simulink library "r2dbe_vdif_lib"  (R2012b)
settings: Solver=ode45  StartTime=0.0  StopTime=10.0  RelTol=1e-3
libraries: xbsIndex_r4 x360, casper_library_delays x11, casper_library_flow_control x3
(part 2 of 4)

== system r2dbe_vdif_lib/vdif/little_end ==
  sim_1 : Inport
  io_delay : xbsIndex_r4/Delay  rst=off  infoeditControl=Selection of Reset will increase slice count due to use of real FFs and instead of SRLs  en=off  latency=0  dbl_ovrd=off  reg_retiming=on  block_type=delay
  r2dbe_10gbe_f_vdif_little_end_user_data_out : xbsIndex_r4/Gateway In  gui_display_data_type=Fixed-point  arith_type=Unsigned  n_bits=32  bin_pt=0  preci_type=Single  exp_width=8  frac_width=24  quantization="Round  (unbiased: +/- Inf)"  overflow=Saturate  period=1  dbl_ovrd=off  timing_constraint=None  locs_specified=off  LOCs={}  UseAsADC=off  ADCChannel='1'  inherit_from_input=off  hdl_port=on  block_type=gatewayin
  reint1 : xbsIndex_r4/Reinterpret  force_arith_type=on  arith_type=Unsigned  force_bin_pt=on  bin_pt=0  block_type=reinterpret
  slice_reg : xbsIndex_r4/Slice  nbits=32  boolean_output=off  mode=Lower Bit Location + Width  bit1=0  base1=MSB of Input  bit0=0  base0=LSB of Input  dbl_ovrd=off  block_type=slice
  in_reg : Outport
  wires:
  reint1/1 -> in_reg/1
  slice_reg/1 -> reint1/1
  io_delay/1 -> slice_reg/1
  sim_1/1 -> r2dbe_10gbe_f_vdif_little_end_user_data_out/1
  r2dbe_10gbe_f_vdif_little_end_user_data_out/1 -> io_delay/1

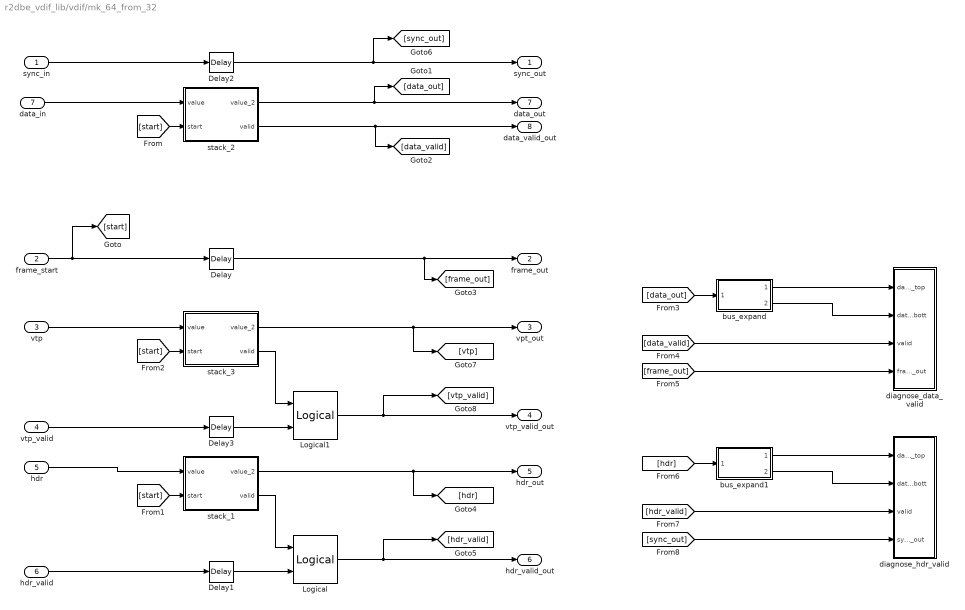
== system r2dbe_vdif_lib/vdif/mk_64_from_32 ==
  sync_in : Inport
  frame_start : Inport  Port=2
  vtp : Inport  Port=3
  vtp_valid : Inport  Port=4
  hdr : Inport  Port=5
  hdr_valid : Inport  Port=6
  data_in : Inport  Port=7
  Delay{,1..3} (4 alike) : xbsIndex_r4/Delay  rst=off  infoeditControl=Selection of Reset will increase slice count due to use of real FFs and instead of SRLs  en=off  latency=2  dbl_ovrd=off  reg_retiming=off  block_type=delay
  Logical : xbsIndex_r4/Logical  logical_function=AND  inputs=2  en=off  latency=0  precision=Full  arith_type=Unsigned  n_bits=16  bin_pt=0  align_bp=on  dbl_ovrd=off  block_type=logical
  Logical1 : xbsIndex_r4/Logical  logical_function=AND  inputs=2  en=off  latency=0  precision=Full  arith_type=Unsigned  n_bits=16  bin_pt=0  align_bp=on  dbl_ovrd=off  block_type=logical
  bus_expand : Subsystem  AncestorBlock=casper_library_flow_control/bus_expand  mask(bus_expand){mode=divisions of equal size, outputNum=2, outputWidth=32, outputBinaryPt=0, outputArithmeticType=0, show_format=off, outputToWorkspace=off, variablePrefix=out, outputToModelAsWell=on}
      mask prompts: outputNum "Number of outputs:"; outputWidth "Output width:"; outputBinaryPt "Output binary point position:"; outputArithmeticType "Output arithmetic type (ufix=0, fix=1, bool=2):"; show_format "Print format string?"; outputToWorkspace "Output to workspace?"; variablePrefix "Variable name prefix:"; outputToModelAsWell "Output to model as well?"
      mask help:
      | Expands a 'bus' made using a bus_create or Xilinx
      | concat block.
      | The input will be divided into the specified number
      | of outputs with the specified arithmetic types.
      | Divisions are made from most significant bit.
      mask init: same as r2dbe_vdif_lib/vdif/delay_data/bus_expand
      settings: AttributesFormatString=2 outputs
      mask TypeOptions mode: divisions of equal size | divisions of arbitrary size
      mask Callback mode: bus_expand_callback();
      mask Callback outputWidth: bus_expand_callback();
      mask Callback outputToWorkspace: bus_expand_callback();
  bus_expand1 : Subsystem  AncestorBlock=casper_library_flow_control/bus_expand  mask(bus_expand){mode=divisions of equal size, outputNum=2, outputWidth=32, outputBinaryPt=0, outputArithmeticType=0, show_format=off, outputToWorkspace=off, variablePrefix=out, outputToModelAsWell=on}
      mask prompts: outputNum "Number of outputs:"; outputWidth "Output width:"; outputBinaryPt "Output binary point position:"; outputArithmeticType "Output arithmetic type (ufix=0, fix=1, bool=2):"; show_format "Print format string?"; outputToWorkspace "Output to workspace?"; variablePrefix "Variable name prefix:"; outputToModelAsWell "Output to model as well?"
      mask help:
      | Expands a 'bus' made using a bus_create or Xilinx
      | concat block.
      | The input will be divided into the specified number
      | of outputs with the specified arithmetic types.
      | Divisions are made from most significant bit.
      mask init: same as r2dbe_vdif_lib/vdif/delay_data/bus_expand
      settings: AttributesFormatString=2 outputs
      mask TypeOptions mode: divisions of equal size | divisions of arbitrary size
      mask Callback mode: bus_expand_callback();
      mask Callback outputWidth: bus_expand_callback();
      mask Callback outputToWorkspace: bus_expand_callback();
  diagnose_data_valid : Subsystem
  diagnose_hdr_valid : Subsystem
  stack_1 : Subsystem
      mask help: stacks 2 samples together, based on a flag that indicates the start or the first sample of data to be stacked. outputs the stacked data and a valid signal, such that on any given valid signal the data represents the newest data in the top half and the oldest data in the lower half. Therefore given a data stream starting with 0, increasing by 1 every clock cycle I would expect the first data valid to indicate a piece of data with the value 0 in the low bits, 1 in the high, and the next sample having 2 in the low bits 3 in the high, etc.
  stack_2 : Subsystem
      mask help: stacks 2 samples together, based on a flag that indicates the start or the first sample of data to be stacked. outputs the stacked data and a valid signal, such that on any given valid signal the data represents the newest data in the top half and the oldest data in the lower half. Therefore given a data stream starting with 0, increasing by 1 every clock cycle I would expect the first data valid to indicate a piece of data with the value 0 in the low bits, 1 in the high, and the next sample having 2 in the low bits 3 in the high, etc.
  stack_3 : Subsystem
      mask help: stacks 2 samples together, based on a flag that indicates the start or the first sample of data to be stacked. outputs the stacked data and a valid signal, such that on any given valid signal the data represents the newest data in the top half and the oldest data in the lower half. Therefore given a data stream starting with 0, increasing by 1 every clock cycle I would expect the first data valid to indicate a piece of data with the value 0 in the low bits, 1 in the high, and the next sample having 2 in the low bits 3 in the high, etc.
  sync_out : Outport
  frame_out : Outport  Port=2
  vpt_out : Outport  Port=3
  vtp_valid_out : Outport  Port=4
  hdr_out : Outport  Port=5
  hdr_valid_out : Outport  Port=6
  data_out : Outport  Port=7
  data_valid_out : Outport  Port=8
  wires:
  hdr_valid/1 -> Delay1/1
  hdr/1 -> stack_1/1(value)
  vtp_valid/1 -> Delay3/1
  vtp/1 -> stack_3/1(value)
  Delay3/1 -> Logical1/2
  Logical1/1 -> [vtp_valid], vtp_valid_out/1
  stack_3/2(valid) -> Logical1/1
  stack_3/1(value_2) -> [vtp], vpt_out/1
  [start] -> stack_3/2(start)
  Delay2/1 -> sync_out/1, [sync_out]
  Delay1/1 -> Logical/2
  Logical/1 -> [hdr_valid], hdr_valid_out/1
  [hdr] -> bus_expand1/1(bus_in)
  [sync_out] -> diagnose_hdr_valid/4(sync_out)
  [hdr_valid] -> diagnose_hdr_valid/3(valid)
  bus_expand1/1(msb_out2) -> diagnose_hdr_valid/1(data_top)
  bus_expand1/2(lsb_out1) -> diagnose_hdr_valid/2(data_bott)
  [data_out] -> bus_expand/1(bus_in)
  [frame_out] -> diagnose_data_valid/4(frame_start_out)
  [data_valid] -> diagnose_data_valid/3(valid)
  bus_expand/1(msb_out2) -> diagnose_data_valid/1(data_top)
  bus_expand/2(lsb_out1) -> diagnose_data_valid/2(data_bott)
  Delay/1 -> frame_out/1, [frame_out]
  stack_1/2(valid) -> Logical/1
  stack_1/1(value_2) -> [hdr], hdr_out/1
  [start] -> stack_1/2(start)
  stack_2/2(valid) -> [data_valid], data_valid_out/1
  stack_2/1(value_2) -> [data_out], data_out/1
  sync_in/1 -> Delay2/1
  [start] -> stack_2/2(start)
  frame_start/1 -> Delay/1, [start]
  data_in/1 -> stack_2/1(value)

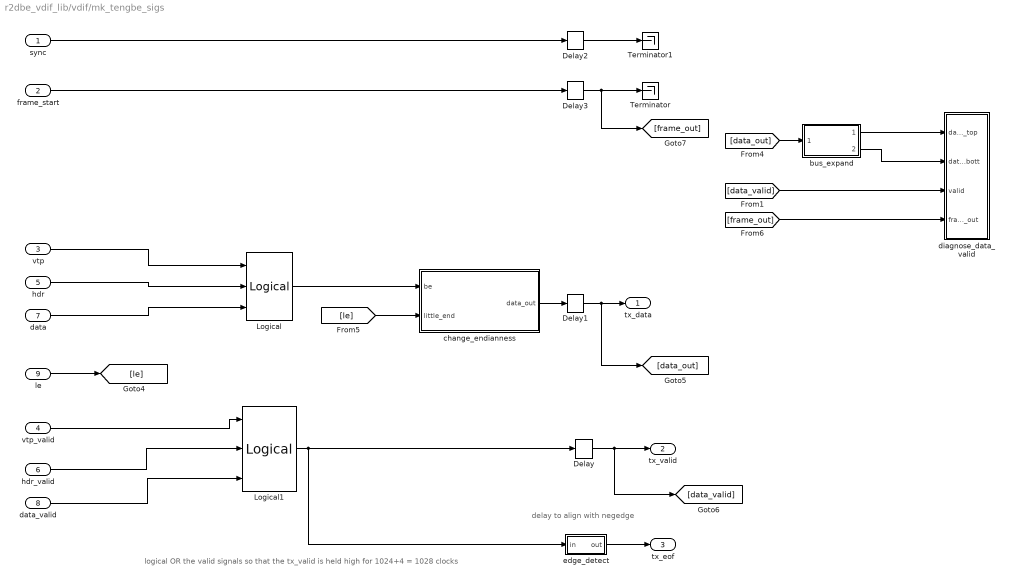
== system r2dbe_vdif_lib/vdif/mk_tengbe_sigs ==
  note: delay to align with
      | negedge
  note: logical OR the valid signals so that the
      | tx_valid is held high for 1024+4 = 1028 clocks
  sync : Inport
  frame_start : Inport  Port=2
  vtp : Inport  Port=3
  vtp_valid : Inport  Port=4
  hdr : Inport  Port=5
  hdr_valid : Inport  Port=6
  data : Inport  Port=7
  data_valid : Inport  Port=8
  le : Inport  Port=9
  Delay{,1..3} (4 alike) : xbsIndex_r4/Delay  rst=off  infoeditControl=Selection of Reset will increase slice count due to use of real FFs and instead of SRLs  en=off  latency=1  dbl_ovrd=off  reg_retiming=off  block_type=delay
  Logical : xbsIndex_r4/Logical  logical_function=XOR  inputs=3  en=off  latency=0  precision=Full  arith_type=Unsigned  n_bits=16  bin_pt=0  align_bp=on  dbl_ovrd=off  block_type=logical
  Logical1 : xbsIndex_r4/Logical  logical_function=XOR  inputs=3  en=off  latency=0  precision=Full  arith_type=Unsigned  n_bits=16  bin_pt=0  align_bp=on  dbl_ovrd=off  block_type=logical
  Terminator : Terminator
  Terminator1 : Terminator
  bus_expand : Subsystem  AncestorBlock=casper_library_flow_control/bus_expand  mask(bus_expand){mode=divisions of equal size, outputNum=2, outputWidth=32, outputBinaryPt=0, outputArithmeticType=0, show_format=off, outputToWorkspace=off, variablePrefix=out, outputToModelAsWell=on}
      mask prompts: outputNum "Number of outputs:"; outputWidth "Output width:"; outputBinaryPt "Output binary point position:"; outputArithmeticType "Output arithmetic type (ufix=0, fix=1, bool=2):"; show_format "Print format string?"; outputToWorkspace "Output to workspace?"; variablePrefix "Variable name prefix:"; outputToModelAsWell "Output to model as well?"
      mask help:
      | Expands a 'bus' made using a bus_create or Xilinx
      | concat block.
      | The input will be divided into the specified number
      | of outputs with the specified arithmetic types.
      | Divisions are made from most significant bit.
      mask init: same as r2dbe_vdif_lib/vdif/delay_data/bus_expand
      settings: AttributesFormatString=2 outputs
      mask TypeOptions mode: divisions of equal size | divisions of arbitrary size
      mask Callback mode: bus_expand_callback();
      mask Callback outputWidth: bus_expand_callback();
      mask Callback outputToWorkspace: bus_expand_callback();
  change_endianness : Subsystem
  diagnose_data_valid : Subsystem
  edge_detect : Subsystem  AncestorBlock=casper_library_misc/edge_detect  mask(edge_detect){edge=Falling, polarity=Active High, x_in=[0 0.08 0.08 0.16 0.16 0.24 0.24 0.32 0.32 0.4], y_in=[-1 -1  1  1  1  1  1  1  1  1], x_out=[0.6 0.68 0.68 0.76 0.76 0.84 0.84 0.92 0.92 1], y_out=[-1 -1  1  1 -1 -1 -1 -1 -1 -1]}
      mask prompts: edge "Edge Type"; polarity "Output Polarity"; x_in "Input X Positions"; y_in "Input Y Positions"; x_out "Output X Positions"; y_out "Output Y Positions"
      mask help: Output is active for one-cycle after each edge of the specified type (i.e. rising, falling or both).
      mask init:
      | edge_detect_init(gcb,...
      |     'edge',edge,...
      |     'polarity',polarity,...
      |     'x_in',x_in,...
      |     'x_out',x_out,...
      |     'y_in',y_in,...
      |     'y_out',y_out);
      | 
      | x_in_num=str2num(getfield(getfield(get_param(gcb,'UserData'),'parameters'),'x_in'));
      | x_out_num=str2num(getfield(getfield(get_param(gcb,'UserData'),'parameters'),'x_out'));
      | y_in_num=str2num(getfield(getfield(get_param(gcb,'UserData'),'parameters'),'y_in'));
      | y_out_num=str2num(getfield(getfield(get_param(gcb,'UserData'),'parameters'),'y_out'));
      settings: AttributesFormatString=|
      | falling edges
      | active high
      mask Help: Output is active for one-cycle after each edge of the specified type (i.e. rising, falling, or both).  Latency is zero.
      mask TypeOptions edge: Rising | Falling | Both
      mask TypeOptions polarity: Active High | Active Low
      mask Display:
      | plot(x_in_num,0.5+y_in_num*0.2);
      | plot(x_out_num,0.5+y_out_num*0.2);
  tx_data : Outport
  tx_valid : Outport  Port=2
  tx_eof : Outport  Port=3
  wires:
  data_valid/1 -> Logical1/3
  hdr_valid/1 -> Logical1/2
  vtp_valid/1 -> Logical1/1
  le/1 -> [le]
  data/1 -> Logical/3
  vtp/1 -> Logical/1
  hdr/1 -> Logical/2
  [data_out] -> bus_expand/1(bus_in)
  [frame_out] -> diagnose_data_valid/4(frame_start_out)
  [data_valid] -> diagnose_data_valid/3(valid)
  bus_expand/1(msb_out2) -> diagnose_data_valid/1(data_top)
  bus_expand/2(lsb_out1) -> diagnose_data_valid/2(data_bott)
  Delay3/1 -> Terminator/1, [frame_out]
  frame_start/1 -> Delay3/1
  Delay1/1 -> tx_data/1, [data_out]
  sync/1 -> Delay2/1
  Delay2/1 -> Terminator1/1
  [le] -> change_endianness/2(little_end)
  change_endianness/1(data_out) -> Delay1/1
  Logical/1 -> change_endianness/1(be)
  Delay/1 -> tx_valid/1, [data_valid]
  Logical1/1 -> Delay/1, edge_detect/1(in)
  edge_detect/1(out) -> tx_eof/1

== system r2dbe_vdif_lib/vdif/reorder ==
  d_native : Inport
  Concat : xbsIndex_r4/Concat  num_inputs=16  dbl_ovrd=off  block_type=concat
  Subsystem : Subsystem
  d_ordered : Outport
  wires:
  Subsystem/16(lsb_out1) -> Concat/1
  Subsystem/15(out2) -> Concat/2
  Subsystem/14(out3) -> Concat/3
  Subsystem/13(out4) -> Concat/4
  Subsystem/12(out5) -> Concat/5
  Subsystem/11(out6) -> Concat/6
  Subsystem/10(out7) -> Concat/7
  Subsystem/9(out8) -> Concat/8
  Subsystem/8(out9) -> Concat/9
  Subsystem/7(out10) -> Concat/10
  Subsystem/6(out11) -> Concat/11
  Subsystem/5(out12) -> Concat/12
  Subsystem/4(out13) -> Concat/13
  Subsystem/3(out14) -> Concat/14
  Subsystem/2(out15) -> Concat/15
  Subsystem/1(msb_out16) -> Concat/16
  d_native/1 -> Subsystem/1(bus_in)
  Concat/1 -> d_ordered/1

== system r2dbe_vdif_lib/vdif/reorder_2b_samps ==
  sim_1 : Inport
  io_delay : xbsIndex_r4/Delay  rst=off  infoeditControl=Selection of Reset will increase slice count due to use of real FFs and instead of SRLs  en=off  latency=0  dbl_ovrd=off  reg_retiming=on  block_type=delay
  r2dbe_10gbe_f_vdif_reorder_2b_samps_user_data_out : xbsIndex_r4/Gateway In  gui_display_data_type=Fixed-point  arith_type=Unsigned  n_bits=32  bin_pt=0  preci_type=Single  exp_width=8  frac_width=24  quantization="Round  (unbiased: +/- Inf)"  overflow=Saturate  period=1  dbl_ovrd=off  timing_constraint=None  locs_specified=off  LOCs={}  UseAsADC=off  ADCChannel='1'  inherit_from_input=off  hdl_port=on  block_type=gatewayin
  reint1 : xbsIndex_r4/Reinterpret  force_arith_type=on  arith_type=Unsigned  force_bin_pt=on  bin_pt=0  block_type=reinterpret
  slice_reg : xbsIndex_r4/Slice  nbits=32  boolean_output=off  mode=Lower Bit Location + Width  bit1=0  base1=MSB of Input  bit0=0  base0=LSB of Input  dbl_ovrd=off  block_type=slice
  in_reg : Outport
  wires:
  reint1/1 -> in_reg/1
  slice_reg/1 -> reint1/1
  io_delay/1 -> slice_reg/1
  sim_1/1 -> r2dbe_10gbe_f_vdif_reorder_2b_samps_user_data_out/1
  r2dbe_10gbe_f_vdif_reorder_2b_samps_user_data_out/1 -> io_delay/1

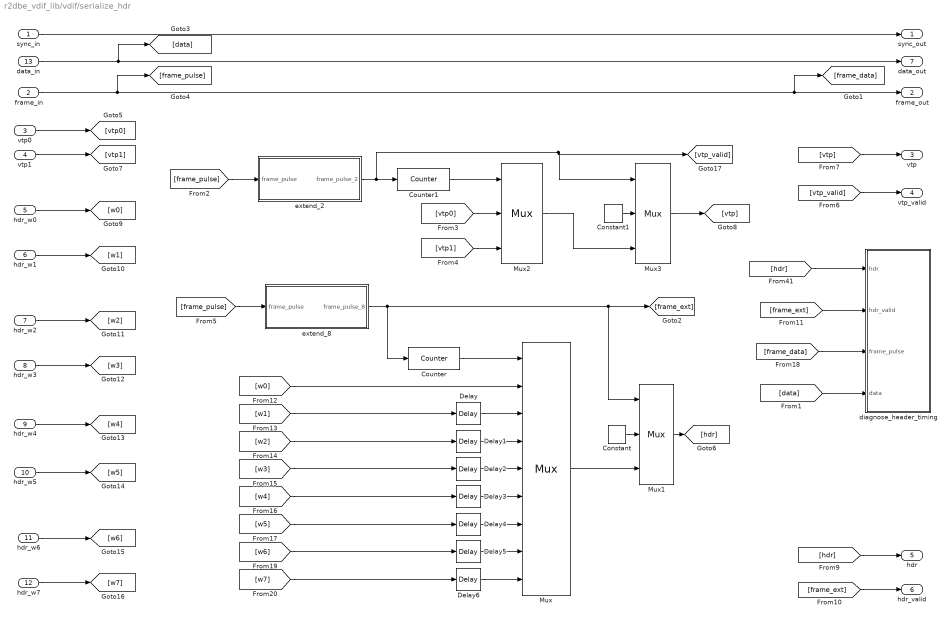
== system r2dbe_vdif_lib/vdif/serialize_hdr ==
  sync_in : Inport
  frame_in : Inport  Port=2
  vtp0 : Inport  Port=3
  vtp1 : Inport  Port=4
  " hdr_w0" : Inport  Port=5
  " hdr_w1" : Inport  Port=6
  " hdr_w2" : Inport  Port=7
  " hdr_w3" : Inport  Port=8
  " hdr_w4" : Inport  Port=9
  " hdr_w5" : Inport  Port=10
  " hdr_w6" : Inport  Port=11
  " hdr_w7" : Inport  Port=12
  " data_in" : Inport  Port=13
  Constant : xbsIndex_r4/Constant  const=0  gui_display_data_type=Fixed-point  arith_type=Unsigned  n_bits=32  bin_pt=0  preci_type=Single  exp_width=8  frac_width=24  explicit_period=on  period=1  equ=P=C  opselect=C  inp2=PCIN>>17  opr=+  inp1=P  carry=CIN  dbl_ovrd=off  block_type=constant
  Constant1 : xbsIndex_r4/Constant  const=0  gui_display_data_type=Fixed-point  arith_type=Unsigned  n_bits=32  bin_pt=0  preci_type=Single  exp_width=8  frac_width=24  explicit_period=on  period=1  equ=P=C  opselect=C  inp2=PCIN>>17  opr=+  inp1=P  carry=CIN  dbl_ovrd=off  block_type=constant
  Counter : xbsIndex_r4/Counter  cnt_type=Free Running  cnt_to=Inf  operation=Up  start_count=0  cnt_by_val=1  arith_type=Unsigned  n_bits=3  bin_pt=0  load_pin=off  rst=off  en=on  explicit_period=on  period=1  dbl_ovrd=off  use_behavioral_HDL=off  implementation=Fabric  block_type=counter
  Counter1 : xbsIndex_r4/Counter  cnt_type=Free Running  cnt_to=Inf  operation=Up  start_count=0  cnt_by_val=1  arith_type=Unsigned  n_bits=1  bin_pt=0  load_pin=off  rst=off  en=on  explicit_period=on  period=1  dbl_ovrd=off  use_behavioral_HDL=off  implementation=Fabric  block_type=counter
  Delay : xbsIndex_r4/Delay  rst=off  infoeditControl=Selection of Reset will increase slice count due to use of real FFs and instead of SRLs  en=off  latency=1  dbl_ovrd=off  reg_retiming=off  block_type=delay
  Delay1 : xbsIndex_r4/Delay  rst=off  infoeditControl=Selection of Reset will increase slice count due to use of real FFs and instead of SRLs  en=off  latency=2  dbl_ovrd=off  reg_retiming=off  block_type=delay
  Delay2 : xbsIndex_r4/Delay  rst=off  infoeditControl=Selection of Reset will increase slice count due to use of real FFs and instead of SRLs  en=off  latency=3  dbl_ovrd=off  reg_retiming=off  block_type=delay
  Delay3 : xbsIndex_r4/Delay  rst=off  infoeditControl=Selection of Reset will increase slice count due to use of real FFs and instead of SRLs  en=off  latency=4  dbl_ovrd=off  reg_retiming=off  block_type=delay
  Delay4 : xbsIndex_r4/Delay  rst=off  infoeditControl=Selection of Reset will increase slice count due to use of real FFs and instead of SRLs  en=off  latency=5  dbl_ovrd=off  reg_retiming=off  block_type=delay
  Delay5 : xbsIndex_r4/Delay  rst=off  infoeditControl=Selection of Reset will increase slice count due to use of real FFs and instead of SRLs  en=off  latency=6  dbl_ovrd=off  reg_retiming=off  block_type=delay
  Delay6 : xbsIndex_r4/Delay  rst=off  infoeditControl=Selection of Reset will increase slice count due to use of real FFs and instead of SRLs  en=off  latency=7  dbl_ovrd=off  reg_retiming=off  block_type=delay
  Mux : xbsIndex_r4/Mux  inputs=8  en=off  latency=0  precision=Full  arith_type=Unsigned  n_bits=16  bin_pt=14  quantization=Truncate  overflow=Wrap  dbl_ovrd=off  block_type=mux
  Mux1 : xbsIndex_r4/Mux  inputs=2  en=off  latency=0  precision=Full  arith_type=Unsigned  n_bits=16  bin_pt=14  quantization=Truncate  overflow=Wrap  dbl_ovrd=off  block_type=mux
  Mux2 : xbsIndex_r4/Mux  inputs=2  en=off  latency=0  precision=Full  arith_type=Unsigned  n_bits=16  bin_pt=14  quantization=Truncate  overflow=Wrap  dbl_ovrd=off  block_type=mux
  Mux3 : xbsIndex_r4/Mux  inputs=2  en=off  latency=0  precision=Full  arith_type=Unsigned  n_bits=16  bin_pt=14  quantization=Truncate  overflow=Wrap  dbl_ovrd=off  block_type=mux
  diagnose_header_timing : Subsystem
  extend_2 : Subsystem
  extend_8 : Subsystem
  sync_out : Outport
  frame_out : Outport  Port=2
  vtp : Outport  Port=3
  vtp_valid : Outport  Port=4
  hdr : Outport  Port=5
  hdr_valid : Outport  Port=6
  data_out : Outport  Port=7
  wires:
  [vtp_valid] -> vtp_valid/1
  [vtp] -> vtp/1
  Mux3/1 -> [vtp]
  [vtp1] -> Mux2/3
  [vtp0] -> Mux2/2
  Mux2/1 -> Mux3/3
  Constant1/1 -> Mux3/2
  Counter1/1 -> Mux2/1
  extend_2/1(frame_pulse_2) -> Counter1/1, Mux3/1, [vtp_valid]
  [frame_pulse] -> extend_2/1(frame_pulse)
  vtp1/1 -> [vtp1]
  vtp0/1 -> [vtp0]
  Constant/1 -> Mux1/2
  Mux/1 -> Mux1/3
  Mux1/1 -> [hdr]
  [data] -> diagnose_header_timing/4(data)
  [w7] -> Delay6/1
  [w6] -> Delay5/1
  [w5] -> Delay4/1
  [w4] -> Delay3/1
  [w3] -> Delay2/1
  [w2] -> Delay1/1
  [w1] -> Delay/1
  [w0] -> Mux/2
  [frame_ext] -> hdr_valid/1
  [hdr] -> hdr/1
  extend_8/1(frame_pulse_8) -> [frame_ext], Mux1/1, Counter/1
  [frame_pulse] -> extend_8/1(frame_pulse)
  Counter/1 -> Mux/1
  Delay6/1 -> Mux/9
  Delay5/1 -> Mux/8
  Delay4/1 -> Mux/7
  Delay3/1 -> Mux/6
  Delay2/1 -> Mux/5
  Delay1/1 -> Mux/4
  Delay/1 -> Mux/3
  frame_in/1 -> frame_out/1, [frame_data], [frame_pulse]
  " data_in"/1 -> [data], data_out/1
  sync_in/1 -> sync_out/1
  " hdr_w7"/1 -> [w7]
  " hdr_w6"/1 -> [w6]
  " hdr_w5"/1 -> [w5]
  " hdr_w4"/1 -> [w4]
  " hdr_w3"/1 -> [w3]
  " hdr_w2"/1 -> [w2]
  " hdr_w1"/1 -> [w1]
  " hdr_w0"/1 -> [w0]
  [hdr] -> diagnose_header_timing/1(hdr)
  [frame_ext] -> diagnose_header_timing/2(hdr_valid)
  [frame_data] -> diagnose_header_timing/3(frame_pulse)

== system r2dbe_vdif_lib/vdif/test_sel ==
  sim_1 : Inport
  io_delay : xbsIndex_r4/Delay  rst=off  infoeditControl=Selection of Reset will increase slice count due to use of real FFs and instead of SRLs  en=off  latency=0  dbl_ovrd=off  reg_retiming=on  block_type=delay
  r2dbe_10gbe_f_vdif_test_sel_user_data_out : xbsIndex_r4/Gateway In  gui_display_data_type=Fixed-point  arith_type=Unsigned  n_bits=32  bin_pt=0  preci_type=Single  exp_width=8  frac_width=24  quantization="Round  (unbiased: +/- Inf)"  overflow=Saturate  period=1  dbl_ovrd=off  timing_constraint=None  locs_specified=off  LOCs={}  UseAsADC=off  ADCChannel='1'  inherit_from_input=off  hdl_port=on  block_type=gatewayin
  reint1 : xbsIndex_r4/Reinterpret  force_arith_type=on  arith_type=Unsigned  force_bin_pt=on  bin_pt=0  block_type=reinterpret
  slice_reg : xbsIndex_r4/Slice  nbits=32  boolean_output=off  mode=Lower Bit Location + Width  bit1=0  base1=MSB of Input  bit0=0  base0=LSB of Input  dbl_ovrd=off  block_type=slice
  in_reg : Outport
  wires:
  reint1/1 -> in_reg/1
  slice_reg/1 -> reint1/1
  io_delay/1 -> slice_reg/1
  sim_1/1 -> r2dbe_10gbe_f_vdif_test_sel_user_data_out/1
  r2dbe_10gbe_f_vdif_test_sel_user_data_out/1 -> io_delay/1

== system r2dbe_vdif_lib/vdif/buffer_data/diagnose_data_valid ==
  data_top : Inport
  data_bott : Inport  Port=2
  valid : Inport  Port=3
  frame_start_out : Inport  Port=4
  Disregard Subsystem : xbsIndex_r4/Disregard Subsystem  Tag=discardX  block_type=disregard
  Gateway Out{1..4} (4 alike) : xbsIndex_r4/Gateway Out  inherit_from_input=off  hdl_port=on  timing_constraint=None  locs_specified=off  LOCs={}  UseAsDAC=off  DACChannel='1'  block_type=gatewayout
  Scope : Scope  NumInputPorts=4
      settings: TimeRange=1.649420126233963  YMin=6.93637e+12~0.95~-1~-5  YMax=7.66651e+12~1.05~1~5
  wires:
  frame_start_out/1 -> Gateway Out4/1  "tx_valid"
  Gateway Out4/1 -> Scope/4  "frame_start_out"
  Gateway Out3/1 -> Scope/2  "data_bott"
  Gateway Out2/1 -> Scope/1  "data_top"
  data_bott/1 -> Gateway Out3/1  "tx_valid"
  data_top/1 -> Gateway Out2/1  "tx_data"
  valid/1 -> Gateway Out1/1  "tx_valid"
  Gateway Out1/1 -> Scope/3  "valid"

== system r2dbe_vdif_lib/vdif/buffer_data/diagnose_hdr_valid ==
  hdr_top : Inport
  hdr_bott : Inport  Port=2
  valid : Inport  Port=3
  sync_out : Inport  Port=4
  Disregard Subsystem : xbsIndex_r4/Disregard Subsystem  Tag=discardX  block_type=disregard
  Gateway Out{1..4} (4 alike) : xbsIndex_r4/Gateway Out  inherit_from_input=off  hdl_port=on  timing_constraint=None  locs_specified=off  LOCs={}  UseAsDAC=off  DACChannel='1'  block_type=gatewayout
  Scope : Scope  NumInputPorts=4
      settings: TimeRange=1.649420126233963  YMin=6.93637e+12~0.95~-1~-5  YMax=7.66651e+12~1.05~1~5
  wires:
  Gateway Out1/1 -> Scope/3  "valid"
  valid/1 -> Gateway Out1/1  "tx_valid"
  hdr_top/1 -> Gateway Out2/1  "tx_data"
  hdr_bott/1 -> Gateway Out3/1  "tx_valid"
  Gateway Out2/1 -> Scope/1  "hdr_top"
  Gateway Out3/1 -> Scope/2  "hdr_bott"
  Gateway Out4/1 -> Scope/4  "sync_out"
  sync_out/1 -> Gateway Out4/1  "tx_valid"

== system r2dbe_vdif_lib/vdif/buffer_data/diagnose_input_data ==
  input_data_top : Inport
  input_data_bott : Inport  Port=2
  valid : Inport  Port=3
  frame_start_int : Inport  Port=4
  Disregard Subsystem : xbsIndex_r4/Disregard Subsystem  Tag=discardX  block_type=disregard
  Gateway Out{1..4} (4 alike) : xbsIndex_r4/Gateway Out  inherit_from_input=off  hdl_port=on  timing_constraint=None  locs_specified=off  LOCs={}  UseAsDAC=off  DACChannel='1'  block_type=gatewayout
  Scope : Scope  NumInputPorts=4
      settings: TimeRange=1.649420126233963  YMin=6.93637e+12~0.95~-1~-5  YMax=7.66651e+12~1.05~1~5
  wires:
  Gateway Out1/1 -> Scope/3  "valid"
  valid/1 -> Gateway Out1/1  "tx_valid"
  input_data_top/1 -> Gateway Out2/1  "tx_data"
  input_data_bott/1 -> Gateway Out3/1  "tx_valid"
  Gateway Out2/1 -> Scope/1  "input_data_top"
  Gateway Out3/1 -> Scope/2  "input_data_bott"
  Gateway Out4/1 -> Scope/4  "frame_start_out"
  frame_start_int/1 -> Gateway Out4/1  "tx_valid"

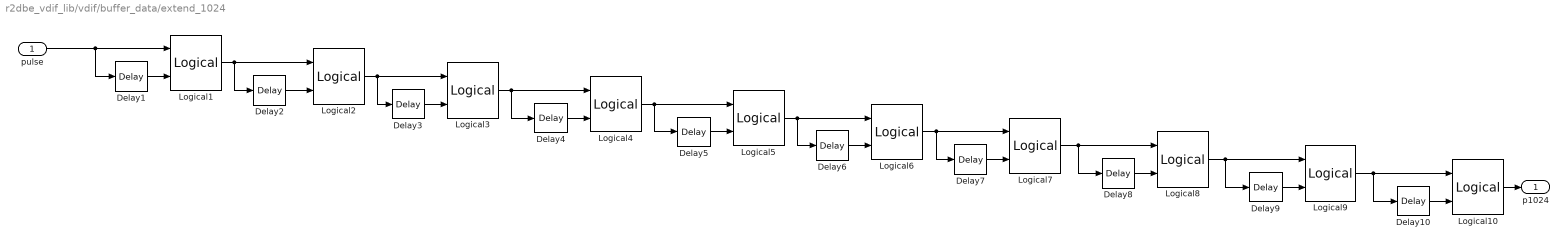
== system r2dbe_vdif_lib/vdif/buffer_data/extend_1024 ==
  pulse : Inport
  Delay1 : xbsIndex_r4/Delay  rst=off  infoeditControl=Selection of Reset will increase slice count due to use of real FFs and instead of SRLs  en=off  latency=1  dbl_ovrd=off  reg_retiming=off  block_type=delay
  Delay10 : xbsIndex_r4/Delay  rst=off  infoeditControl=Selection of Reset will increase slice count due to use of real FFs and instead of SRLs  en=off  latency=512  dbl_ovrd=off  reg_retiming=off  block_type=delay
  Delay2 : xbsIndex_r4/Delay  rst=off  infoeditControl=Selection of Reset will increase slice count due to use of real FFs and instead of SRLs  en=off  latency=2  dbl_ovrd=off  reg_retiming=off  block_type=delay
  Delay3 : xbsIndex_r4/Delay  rst=off  infoeditControl=Selection of Reset will increase slice count due to use of real FFs and instead of SRLs  en=off  latency=4  dbl_ovrd=off  reg_retiming=off  block_type=delay
  Delay4 : xbsIndex_r4/Delay  rst=off  infoeditControl=Selection of Reset will increase slice count due to use of real FFs and instead of SRLs  en=off  latency=8  dbl_ovrd=off  reg_retiming=off  block_type=delay
  Delay5 : xbsIndex_r4/Delay  rst=off  infoeditControl=Selection of Reset will increase slice count due to use of real FFs and instead of SRLs  en=off  latency=16  dbl_ovrd=off  reg_retiming=off  block_type=delay
  Delay6 : xbsIndex_r4/Delay  rst=off  infoeditControl=Selection of Reset will increase slice count due to use of real FFs and instead of SRLs  en=off  latency=32  dbl_ovrd=off  reg_retiming=off  block_type=delay
  Delay7 : xbsIndex_r4/Delay  rst=off  infoeditControl=Selection of Reset will increase slice count due to use of real FFs and instead of SRLs  en=off  latency=64  dbl_ovrd=off  reg_retiming=off  block_type=delay
  Delay8 : xbsIndex_r4/Delay  rst=off  infoeditControl=Selection of Reset will increase slice count due to use of real FFs and instead of SRLs  en=off  latency=128  dbl_ovrd=off  reg_retiming=off  block_type=delay
  Delay9 : xbsIndex_r4/Delay  rst=off  infoeditControl=Selection of Reset will increase slice count due to use of real FFs and instead of SRLs  en=off  latency=256  dbl_ovrd=off  reg_retiming=off  block_type=delay
  Logical{1..10} (10 alike) : xbsIndex_r4/Logical  logical_function=OR  inputs=2  en=off  latency=0  precision=Full  arith_type=Unsigned  n_bits=16  bin_pt=0  align_bp=on  dbl_ovrd=off  block_type=logical
  p1024 : Outport
  wires:
  Logical10/1 -> p1024/1
  Delay10/1 -> Logical10/2
  Logical9/1 -> Logical10/1, Delay10/1
  Delay9/1 -> Logical9/2
  Logical8/1 -> Delay9/1, Logical9/1
  Delay8/1 -> Logical8/2
  Logical7/1 -> Logical8/1, Delay8/1
  Delay7/1 -> Logical7/2
  Logical6/1 -> Delay7/1, Logical7/1
  Delay6/1 -> Logical6/2
  Logical5/1 -> Logical6/1, Delay6/1
  Delay5/1 -> Logical5/2
  Logical4/1 -> Delay5/1, Logical5/1
  Delay4/1 -> Logical4/2
  Logical3/1 -> Logical4/1, Delay4/1
  Delay3/1 -> Logical3/2
  Logical2/1 -> Logical3/1, Delay3/1
  pulse/1 -> Delay1/1, Logical1/1
  Delay1/1 -> Logical1/2
  Logical1/1 -> Delay2/1, Logical2/1
  Delay2/1 -> Logical2/2

== system r2dbe_vdif_lib/vdif/buffer_data/extend_4 ==
  pulse : Inport
  Delay1 : xbsIndex_r4/Delay  rst=off  infoeditControl=Selection of Reset will increase slice count due to use of real FFs and instead of SRLs  en=off  latency=1  dbl_ovrd=off  reg_retiming=off  block_type=delay
  Delay2 : xbsIndex_r4/Delay  rst=off  infoeditControl=Selection of Reset will increase slice count due to use of real FFs and instead of SRLs  en=off  latency=2  dbl_ovrd=off  reg_retiming=off  block_type=delay
  Logical1 : xbsIndex_r4/Logical  logical_function=OR  inputs=2  en=off  latency=0  precision=Full  arith_type=Unsigned  n_bits=16  bin_pt=0  align_bp=on  dbl_ovrd=off  block_type=logical
  Logical2 : xbsIndex_r4/Logical  logical_function=OR  inputs=2  en=off  latency=0  precision=Full  arith_type=Unsigned  n_bits=16  bin_pt=0  align_bp=on  dbl_ovrd=off  block_type=logical
  pulse_4 : Outport
  wires:
  Delay2/1 -> Logical2/2
  Logical1/1 -> Logical2/1, Delay2/1
  Delay1/1 -> Logical1/2
  Logical2/1 -> pulse_4/1
  pulse/1 -> Logical1/1, Delay1/1

== system r2dbe_vdif_lib/vdif/delay_data/bus_expand ==
  bus_in : Inport
  reinterpret1 : xbsIndex_r4/Reinterpret  force_arith_type=on  arith_type=Unsigned  force_bin_pt=on  bin_pt=0  block_type=reinterpret
  reinterpret2 : xbsIndex_r4/Reinterpret  force_arith_type=on  arith_type=Unsigned  force_bin_pt=on  bin_pt=0  block_type=reinterpret
  slice1 : xbsIndex_r4/Slice  nbits=32  boolean_output=off  mode=Upper Bit Location + Width  bit1=-32  base1=MSB of Input  bit0=0  base0=LSB of Input  dbl_ovrd=off  block_type=slice
  slice2 : xbsIndex_r4/Slice  nbits=32  boolean_output=off  mode=Upper Bit Location + Width  bit1=0  base1=MSB of Input  bit0=0  base0=LSB of Input  dbl_ovrd=off  block_type=slice
  msb_out2 : Outport
  lsb_out1 : Outport  Port=2
  wires:
  bus_in/1 -> slice2/1, slice1/1
  slice2/1 -> reinterpret2/1
  reinterpret2/1 -> msb_out2/1
  slice1/1 -> reinterpret1/1
  reinterpret1/1 -> lsb_out1/1

== system r2dbe_vdif_lib/vdif/delay_data/bus_expand1 ==
  bus_in : Inport
  reinterpret1 : xbsIndex_r4/Reinterpret  force_arith_type=on  arith_type=Unsigned  force_bin_pt=on  bin_pt=0  block_type=reinterpret
  reinterpret2 : xbsIndex_r4/Reinterpret  force_arith_type=on  arith_type=Unsigned  force_bin_pt=on  bin_pt=0  block_type=reinterpret
  slice1 : xbsIndex_r4/Slice  nbits=32  boolean_output=off  mode=Upper Bit Location + Width  bit1=-32  base1=MSB of Input  bit0=0  base0=LSB of Input  dbl_ovrd=off  block_type=slice
  slice2 : xbsIndex_r4/Slice  nbits=32  boolean_output=off  mode=Upper Bit Location + Width  bit1=0  base1=MSB of Input  bit0=0  base0=LSB of Input  dbl_ovrd=off  block_type=slice
  msb_out2 : Outport
  lsb_out1 : Outport  Port=2
  wires:
  bus_in/1 -> slice2/1, slice1/1
  slice2/1 -> reinterpret2/1
  reinterpret2/1 -> msb_out2/1
  slice1/1 -> reinterpret1/1
  reinterpret1/1 -> lsb_out1/1

== system r2dbe_vdif_lib/vdif/delay_data/diagnose_data_valid ==
  data_top : Inport
  data_bott : Inport  Port=2
  data_valid : Inport  Port=3
  hdr_top : Inport  Port=4
  hdr_bott : Inport  Port=5
  hdr_valid : Inport  Port=6
  Disregard Subsystem : xbsIndex_r4/Disregard Subsystem  Tag=discardX  block_type=disregard
  Gateway Out{1..6} (6 alike) : xbsIndex_r4/Gateway Out  inherit_from_input=off  hdl_port=on  timing_constraint=None  locs_specified=off  LOCs={}  UseAsDAC=off  DACChannel='1'  block_type=gatewayout
  Scope : Scope  NumInputPorts=6
      settings: TimeRange=1.649420126233963  YMin=6.93637e+12~0.95~-1~-5~-5~-5  YMax=7.66651e+12~1.05~1~5~5~5
  wires:
  Gateway Out6/1 -> Scope/6  "hdr_valid"
  hdr_valid/1 -> Gateway Out6/1
  Gateway Out5/1 -> Scope/5  "hdr_bott"
  hdr_bott/1 -> Gateway Out5/1
  Gateway Out1/1 -> Scope/3  "data_valid"
  data_valid/1 -> Gateway Out1/1  "tx_valid"
  data_top/1 -> Gateway Out2/1  "tx_data"
  data_bott/1 -> Gateway Out3/1  "tx_valid"
  Gateway Out2/1 -> Scope/1  "data_top"
  Gateway Out3/1 -> Scope/2  "data_bott"
  Gateway Out4/1 -> Scope/4  "hdr_top"
  hdr_top/1 -> Gateway Out4/1  "tx_valid"

== system r2dbe_vdif_lib/vdif/delay_data/diagnose_data_valid1 ==
  sync : Inport
  frame : Inport  Port=2
  data_valid : Inport  Port=3
  hdr_valid : Inport  Port=4
  Disregard Subsystem : xbsIndex_r4/Disregard Subsystem  Tag=discardX  block_type=disregard
  Gateway Out{1..4} (4 alike) : xbsIndex_r4/Gateway Out  inherit_from_input=off  hdl_port=on  timing_constraint=None  locs_specified=off  LOCs={}  UseAsDAC=off  DACChannel='1'  block_type=gatewayout
  Scope : Scope  NumInputPorts=4
      settings: TimeRange=1.649420126233963  YMin=6.93637e+12~0.95~-1~-5  YMax=7.66651e+12~1.05~1~5
  wires:
  hdr_valid/1 -> Gateway Out4/1  "tx_valid"
  Gateway Out4/1 -> Scope/4  "hdr_valid"
  Gateway Out3/1 -> Scope/2  "frame_out"
  Gateway Out2/1 -> Scope/1  "sync_out"
  frame/1 -> Gateway Out3/1  "tx_valid"
  sync/1 -> Gateway Out2/1  "tx_data"
  data_valid/1 -> Gateway Out1/1  "tx_valid"
  Gateway Out1/1 -> Scope/3  "data_valid"

== system r2dbe_vdif_lib/vdif/hdr/diagnose_input_timing ==
  sync : Inport
  enable : Inport  Port=2
  start_frame : Inport  Port=3
  data : Inport  Port=4
  Disregard Subsystem : xbsIndex_r4/Disregard Subsystem  Tag=discardX  block_type=disregard
  Gateway Out{,1..3} (4 alike) : xbsIndex_r4/Gateway Out  inherit_from_input=off  hdl_port=on  timing_constraint=None  locs_specified=off  LOCs={}  UseAsDAC=off  DACChannel='1'  block_type=gatewayout
  Scope : Scope  NumInputPorts=4
      settings: TimeRange=1.649420126233963  YMin=2.85~5.25966e+08~-5~-5  YMax=3.15~5.8133e+08~5~5
  wires:
  data/1 -> Gateway Out3/1  "re"
  Gateway Out3/1 -> Scope/4  "data"
  start_frame/1 -> Gateway Out2/1  "re"
  Gateway Out2/1 -> Scope/3  "start_frame"
  sync/1 -> Gateway Out/1  "dout"
  enable/1 -> Gateway Out1/1  "re"
  Gateway Out1/1 -> Scope/2  "en"
  Gateway Out/1 -> Scope/1  "sync"

== system r2dbe_vdif_lib/vdif/hdr/diagnose_input_timing1 ==
  secs : Inport
  frame : Inport  Port=2
  data : Inport  Port=3
  pps : Inport  Port=4
  Disregard Subsystem : xbsIndex_r4/Disregard Subsystem  Tag=discardX  block_type=disregard
  Gateway Out{,1,3..4} (4 alike) : xbsIndex_r4/Gateway Out  inherit_from_input=off  hdl_port=on  timing_constraint=None  locs_specified=off  LOCs={}  UseAsDAC=off  DACChannel='1'  block_type=gatewayout
  Scope : Scope  NumInputPorts=4
      settings: TimeRange=1.649420126233963  YMin=2.85~5.25966e+08~-5~-5  YMax=3.15~5.8133e+08~5~5
  wires:
  Gateway Out3/1 -> Scope/3  "data"
  Gateway Out4/1 -> Scope/4  "pps"
  pps/1 -> Gateway Out4/1  "re"
  Gateway Out/1 -> Scope/1  "secs"
  Gateway Out1/1 -> Scope/2  "frame"
  frame/1 -> Gateway Out1/1  "re"
  secs/1 -> Gateway Out/1  "dout"
  data/1 -> Gateway Out3/1  "re"

== system r2dbe_vdif_lib/vdif/hdr/diagnose_input_timing2 ==
  w6 : Inport
  w7 : Inport  Port=2
  data : Inport  Port=3
  pps : Inport  Port=4
  Disregard Subsystem : xbsIndex_r4/Disregard Subsystem  Tag=discardX  block_type=disregard
  Gateway Out{,1,3..4} (4 alike) : xbsIndex_r4/Gateway Out  inherit_from_input=off  hdl_port=on  timing_constraint=None  locs_specified=off  LOCs={}  UseAsDAC=off  DACChannel='1'  block_type=gatewayout
  Scope : Scope  NumInputPorts=4
      settings: TimeRange=1.649420126233963  YMin=3~5.25966e+08~-5~-5  YMax=3~5.8133e+08~5~5
  wires:
  data/1 -> Gateway Out3/1  "re"
  w6/1 -> Gateway Out/1  "dout"
  w7/1 -> Gateway Out1/1  "re"
  Gateway Out1/1 -> Scope/2  "w7"
  Gateway Out/1 -> Scope/1  "w6"
  pps/1 -> Gateway Out4/1  "re"
  Gateway Out4/1 -> Scope/4  "pps"
  Gateway Out3/1 -> Scope/3  "data"

== system r2dbe_vdif_lib/vdif/hdr/pulse_every_2048 ==
  en : Inport
  Constant : xbsIndex_r4/Constant  const=0  gui_display_data_type=Fixed-point  arith_type=Unsigned  n_bits=1  bin_pt=0  preci_type=Single  exp_width=8  frac_width=24  explicit_period=on  period=1  equ=P=C  opselect=C  inp2=PCIN>>17  opr=+  inp1=P  carry=CIN  dbl_ovrd=off  block_type=constant
  Counter : xbsIndex_r4/Counter  cnt_type=Count Limited  cnt_to=max(per,2)-1  operation=Up  start_count=0  cnt_by_val=1  arith_type=Unsigned  n_bits=nextpow2(max(per,2))  bin_pt=0  load_pin=off  rst=off  en=on  explicit_period=on  period=1  dbl_ovrd=off  use_behavioral_HDL=off  implementation=Fabric  block_type=counter
  Logical : xbsIndex_r4/Logical  logical_function=AND  inputs=2  en=off  latency=0  precision=Full  arith_type=Unsigned  n_bits=16  bin_pt=0  align_bp=on  dbl_ovrd=off  block_type=logical
  Relational : xbsIndex_r4/Relational  mode=a=b  en=off  latency=0  dbl_ovrd=off  block_type=relational
  pulse : Outport
  wires:
  Constant/1 -> Relational/2
  Logical/1 -> pulse/1
  Relational/1 -> Logical/1
  Counter/1 -> Relational/1
  en/1 -> Counter/1, Logical/2

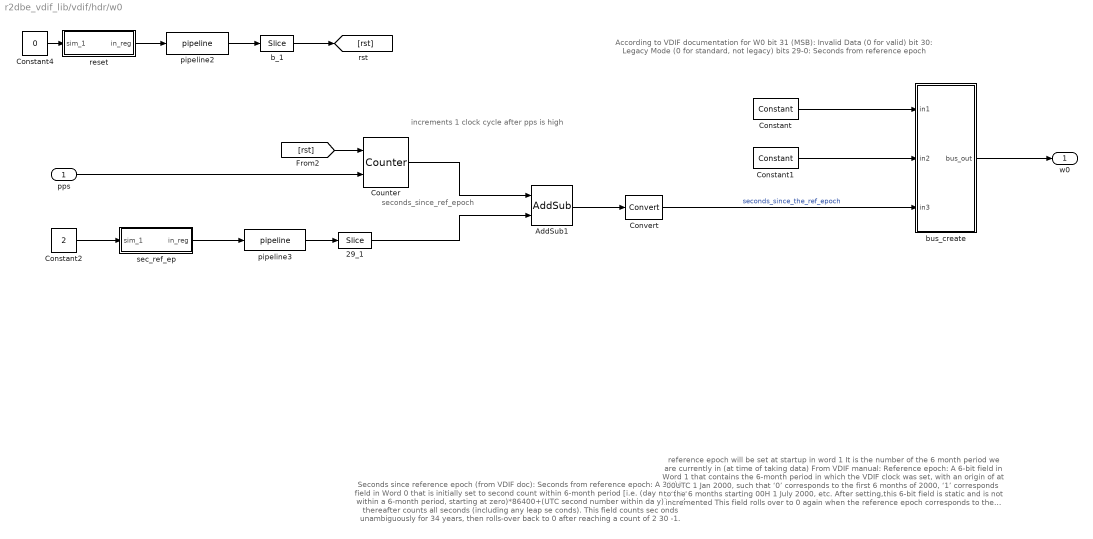
== system r2dbe_vdif_lib/vdif/hdr/w0 ==
  note: Seconds since reference epoch (from VDIF doc):
      |
      | Seconds from reference epoch: A 30-bit field
      | in Word 0 that is initially set to second
      | count within 6-month period
      | [i.e. (day number within a
      | 6-month period, starting at
      | zero)*86400+(UTC second number within da
      | y)], and thereafter counts all
      | seconds
      | (including any leap se
      | conds). This field counts sec
      | onds unambiguously for 34 years,
      | then rolls-over back to 0
      | after reaching a count of 2
      | 30
      | -1.
  note: reference epoch will be set at startup in word 1
      | It is the number of the 6 month period we are currently in (at time of taking data)
      | From VDIF manual:
      |
      |
      | Reference epoch: A 6-bit field in Word 1
      | that contains the 6-month period
      |  in which the VDIF clock was set,
      | with an origin of at 00UTC 1 Jan 2000,
      | such that
      | ‘0’ corresponds to the first 6 months of 2000,
      | ‘1’ corresponds to the 6 months starting
      | 00H 1 July 2000, etc.
      |
      | After setting,this 6-bit field is static and is not incremented
      |
      | This field rolls over to 0 again when
      | the reference epoch corresponds to the 6-month
      | period starting 00H 1 Jan 2032
      |
      |
      | So July 1 - Dec 31 2014 is reference epoch 29?
  note: According to VDIF documentation for W0
      |
      |
      | bit 31 (MSB): Invalid Data (0 for valid)
      | bit 30: Legacy Mode (0 for standard, not legacy)
      |
      |
      |
      | bits 29-0: Seconds from reference epoch
  note: seconds_since_ref_epoch
  note: increments 1 clock cycle after pps is high
  pps : Inport
  29_1 : xbsIndex_r4/Slice  nbits=29  boolean_output=off  mode=Lower Bit Location + Width  bit1=23  base1=LSB of Input  bit0=0  base0=LSB of Input  dbl_ovrd=off  block_type=slice
  AddSub1 : xbsIndex_r4/AddSub  mode=Addition  use_carryin=off  use_carryout=off  en=off  latency=0  precision=Full  arith_type=Unsigned  n_bits=16  bin_pt=14  quantization=Truncate  overflow=Wrap  dbl_ovrd=off  use_behavioral_HDL=off  hw_selection=Fabric  pipelined=off  block_type=addsub
  Constant : xbsIndex_r4/Constant  const=0  gui_display_data_type=Fixed-point  arith_type=Unsigned  n_bits=1  bin_pt=0  preci_type=Single  exp_width=8  frac_width=24  explicit_period=on  period=1  equ=P=C  opselect=C  inp2=PCIN>>17  opr=+  inp1=P  carry=CIN  dbl_ovrd=off  block_type=constant
  Constant1 : xbsIndex_r4/Constant  const=0  gui_display_data_type=Boolean  arith_type=Boolean  n_bits=16  bin_pt=14  preci_type=Single  exp_width=8  frac_width=24  explicit_period=on  period=1  equ=P=C  opselect=C  inp2=PCIN>>17  opr=+  inp1=P  carry=CIN  dbl_ovrd=off  block_type=constant
  Constant2 : Constant  Value=2
  Constant4 : Constant  Value=0
  Convert : xbsIndex_r4/Convert  gui_display_data_type=Fixed-point  arith_type=Unsigned  n_bits=30  bin_pt=0  float_type=Single  exp_bits=8  fraction_bits=24  quantization=Truncate  overflow=Wrap  en=off  latency=0  dbl_ovrd=off  pipeline=off  block_type=convert
  Counter : xbsIndex_r4/Counter  cnt_type=Free Running  cnt_to=Inf  operation=Up  start_count=0  cnt_by_val=1  arith_type=Unsigned  n_bits=29  bin_pt=0  load_pin=off  rst=on  en=on  explicit_period=on  period=1  dbl_ovrd=off  use_behavioral_HDL=off  implementation=Fabric  block_type=counter
  b_1 : xbsIndex_r4/Slice  nbits=1  boolean_output=on  mode=Upper Bit Location + Width  bit1=0  base1=LSB of Input  bit0=0  base0=LSB of Input  dbl_ovrd=off  block_type=slice
  bus_create : Subsystem  mask(bus_create){inputNum=3}
      mask prompts: inputNum "Number of inputs:"
      mask init:
      | bus_create_init(gcb,...
      |     'inputNum', inputNum);
  pipeline2 : casper_library_delays/pipeline  latency=1
      settings: AttributesFormatString=Latency = %<latency>
  pipeline3 : casper_library_delays/pipeline  latency=1
      settings: AttributesFormatString=Latency = %<latency>
  reset : Subsystem  Tag=xps:sw_reg  AncestorBlock=xps_library/software register  mask(swreg){mode=one value, io_dir=From Processor, io_delay=0, sample_period=1, names=reg, bitwidths=32, arith_types=0, bin_pts=0, sim_port=on, show_format=off}
      mask prompts: io_dir "I/O direction"; io_delay "I/O delay"; sample_period "Sample period"; names "Name:"; bitwidths "Bitwidth:"; arith_types "Type (ufix=0, fix=1, bool=2):"; bin_pts "Binary pt:"; sim_port "Provide sim input/output?"; show_format "Print format string?"
      mask init:
      | swreg_init(gcb)
      settings: AttributesFormatString=1input
      mask TypeOptions mode: one value | fields of equal size | fields of arbitrary size
      mask Callback mode: swreg_cb(gcb);
      mask TypeOptions io_dir: To Processor | From Processor
      mask Callback io_dir:
      | mask_enables = get_param(gcb, 'MaskEnables');
      | mask_names = get_param(gcb, 'MaskNames');
      | if strcmp(get_param(gcb, 'io_dir'), 'To Processor'),
      |     mask_enables{ismember(mask_names, 'sample_period')} = 'off';
      | else
      |     mask_enables{ismember(mask_names, 'sample_period')} = 'on';
      | end
      | set_param(gcb, 'MaskEnables', mask_enables);
      mask Callback bitwidths:
      | swreg_maskcheck(gcb);
      | % blk = gcb;
      | % mode = get_param(blk, 'mode');
      | % current_widths = eval(get_param(blk, 'bitwidths'));
      | % if (strcmp(mode, 'one value') || strcmp(mode, 'fields of equal size')) && (length(current_widths) > 1),
      | %     error('Only one width may be specified for this mode.');
      | % elseif strcmp(mode, 'fields of arbitrary size')
      | %     current_names = textscan(strtrim(strrep(strrep(get_param(blk, 'names'), ']', ''), '[', '')), '%s');
      | %     current_names = current_names{1};
      | %     numios = length(current_names);
      | %     if length(current_widths) ~= numios,
      | %         error('%d field names specified, but %d widths?', numios, length(current_widths));
      | %     end
      | % end
      | % total_width = 0;
      | % for ctr = 1 : length(current_widths),
      | %     total_width = total_width + current_widths(ctr);
      | % end
      | % if total_width > 32,
      | %     error('Total width must be 32 or less, set to %d.', total_width);
      | % end
      mask Callback arith_types:
      | [numios, ~, ~, ~, current_types] = swreg_maskcheck(gcb);
      | % blk = gcb;
      | % mode = get_param(blk, 'mode');
      | % current_types = eval(get_param(blk, 'arith_types'));
      | % numios = length(current_types);
      | % if (strcmp(mode, 'one value') || strcmp(mode, 'fields of equal size')) && (length(current_types) > 1),
      | %     error('Only one type may be specified for this mode.');
      | % elseif strcmp(mode, 'fields of arbitrary size')
      | %     current_names = textscan(strtrim(strrep(strrep(get_param(blk, 'names'), ']', ''), '[', '')), '%s');
      | %     current_names = current_names{1};
      | %     numios = length(current_names);
      | %     if length(current_types) ~= numios,
      | %         error('%d field names specified, but %d types?', numios, length(current_types));
      | %     end
      | % end
      | problem = 0;
      | for ctr = 1 : numios,
      |     t = current_types(ctr);
      |     if (t < 0) || (t > 2),
      |         problem = t;
      |         ctr = numios + 1;
      |     end
      | end
      | if problem ~= 0,
      |     error('Type cannot be %i, must be 0, 1 or 2.', problem);
      | end
      mask Callback bin_pts:
      | swreg_maskcheck(gcb);
      | % blk = gcb;
      | % mode = get_param(blk, 'mode');
      | % current_bins = eval(get_param(blk, 'bin_pts'));
      | % if (strcmp(mode, 'one value') || strcmp(mode, 'fields of equal size')) && (length(current_bins) > 1),
      | %     error('Only one binary pt may be specified for this mode.');
      | % elseif strcmp(mode, 'fields of arbitrary size')
      | %     current_names = textscan(strtrim(strrep(strrep(get_param(blk, 'names'), ']', ''), '[', '')), '%s');
      | %     current_names = current_names{1};
      | %     numios = length(current_names);
      | %     if length(current_bins) ~= numios,
      | %         error('%d field names specified, but %d binary pts?', numios, length(current_bins));
      | %     end
      | % end
  sec_ref_ep : Subsystem  Tag=xps:sw_reg  AncestorBlock=xps_library/software register  mask(swreg){mode=one value, io_dir=From Processor, io_delay=0, sample_period=1, names=reg, bitwidths=32, arith_types=0, bin_pts=0, sim_port=on, show_format=off}
      mask prompts: io_dir "I/O direction"; io_delay "I/O delay"; sample_period "Sample period"; names "Name:"; bitwidths "Bitwidth:"; arith_types "Type (ufix=0, fix=1, bool=2):"; bin_pts "Binary pt:"; sim_port "Provide sim input/output?"; show_format "Print format string?"
      mask init:
      | swreg_init(gcb)
      settings: AttributesFormatString=1input
      mask TypeOptions mode: one value | fields of equal size | fields of arbitrary size
      mask Callback mode: swreg_cb(gcb);
      mask TypeOptions io_dir: To Processor | From Processor
      mask Callback io_dir:
      | mask_enables = get_param(gcb, 'MaskEnables');
      | mask_names = get_param(gcb, 'MaskNames');
      | if strcmp(get_param(gcb, 'io_dir'), 'To Processor'),
      |     mask_enables{ismember(mask_names, 'sample_period')} = 'off';
      | else
      |     mask_enables{ismember(mask_names, 'sample_period')} = 'on';
      | end
      | set_param(gcb, 'MaskEnables', mask_enables);
      mask Callback bitwidths:
      | swreg_maskcheck(gcb);
      | % blk = gcb;
      | % mode = get_param(blk, 'mode');
      | % current_widths = eval(get_param(blk, 'bitwidths'));
      | % if (strcmp(mode, 'one value') || strcmp(mode, 'fields of equal size')) && (length(current_widths) > 1),
      | %     error('Only one width may be specified for this mode.');
      | % elseif strcmp(mode, 'fields of arbitrary size')
      | %     current_names = textscan(strtrim(strrep(strrep(get_param(blk, 'names'), ']', ''), '[', '')), '%s');
      | %     current_names = current_names{1};
      | %     numios = length(current_names);
      | %     if length(current_widths) ~= numios,
      | %         error('%d field names specified, but %d widths?', numios, length(current_widths));
      | %     end
      | % end
      | % total_width = 0;
      | % for ctr = 1 : length(current_widths),
      | %     total_width = total_width + current_widths(ctr);
      | % end
      | % if total_width > 32,
      | %     error('Total width must be 32 or less, set to %d.', total_width);
      | % end
      mask Callback arith_types:
      | [numios, ~, ~, ~, current_types] = swreg_maskcheck(gcb);
      | % blk = gcb;
      | % mode = get_param(blk, 'mode');
      | % current_types = eval(get_param(blk, 'arith_types'));
      | % numios = length(current_types);
      | % if (strcmp(mode, 'one value') || strcmp(mode, 'fields of equal size')) && (length(current_types) > 1),
      | %     error('Only one type may be specified for this mode.');
      | % elseif strcmp(mode, 'fields of arbitrary size')
      | %     current_names = textscan(strtrim(strrep(strrep(get_param(blk, 'names'), ']', ''), '[', '')), '%s');
      | %     current_names = current_names{1};
      | %     numios = length(current_names);
      | %     if length(current_types) ~= numios,
      | %         error('%d field names specified, but %d types?', numios, length(current_types));
      | %     end
      | % end
      | problem = 0;
      | for ctr = 1 : numios,
      |     t = current_types(ctr);
      |     if (t < 0) || (t > 2),
      |         problem = t;
      |         ctr = numios + 1;
      |     end
      | end
      | if problem ~= 0,
      |     error('Type cannot be %i, must be 0, 1 or 2.', problem);
      | end
      mask Callback bin_pts:
      | swreg_maskcheck(gcb);
      | % blk = gcb;
      | % mode = get_param(blk, 'mode');
      | % current_bins = eval(get_param(blk, 'bin_pts'));
      | % if (strcmp(mode, 'one value') || strcmp(mode, 'fields of equal size')) && (length(current_bins) > 1),
      | %     error('Only one binary pt may be specified for this mode.');
      | % elseif strcmp(mode, 'fields of arbitrary size')
      | %     current_names = textscan(strtrim(strrep(strrep(get_param(blk, 'names'), ']', ''), '[', '')), '%s');
      | %     current_names = current_names{1};
      | %     numios = length(current_names);
      | %     if length(current_bins) ~= numios,
      | %         error('%d field names specified, but %d binary pts?', numios, length(current_bins));
      | %     end
      | % end
  w0 : Outport
  wires:
  Convert/1 -> bus_create/3(in3)  "seconds_since_the_ref_epoch"
  Constant1/1 -> bus_create/2(in2)
  Constant/1 -> bus_create/1(in1)
  bus_create/1(bus_out) -> w0/1
  AddSub1/1 -> Convert/1
  pps/1 -> Counter/2
  b_1/1 -> [rst]
  Counter/1 -> AddSub1/1
  [rst] -> Counter/1
  Constant4/1 -> reset/1(sim_1)
  reset/1(in_reg) -> pipeline2/1
  pipeline2/1 -> b_1/1
  Constant2/1 -> sec_ref_ep/1(sim_1)
  sec_ref_ep/1(in_reg) -> pipeline3/1
  pipeline3/1 -> 29_1/1
  29_1/1 -> AddSub1/2
